simulink model "x_dd"  (R2020b)
settings: Solver=VariableStepAuto  StartTime=0.0  StopTime=10.0  RelTol=1e-3
settings Model: Creator=64200047  LastModifiedBy=64200047

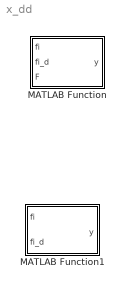
== system x_dd ==
  MATLAB Function : MATLAB Function  TreatAsAtomicUnit=on
  MATLAB Function1 : MATLAB Function  TreatAsAtomicUnit=on

== matlab function x_dd/MATLAB Function ==
  data: fi input; y output; fi_d input; F input
function y = fcn(fi, fi_d, F)
% x 

m1 = 2;
m2 = 0.31;
l = 0.5;

c1 = 1/(m1+m2);
k1 = +m2*l*sin(fi)*fi_d^2;
k2 = m2*l*cos(fi)*(cos(fi) + g*sin(fi));


y = c1*(k1+k2+F);

== matlab function x_dd/MATLAB Function1 ==
  data: fi input; y output; fi_d input
function y = fcn(fi, fi_d)
% fi

m1 = 2;
m2 = 0.31;
l = 0.5;
g = 9.81;

c1 = 1/(-(m2*l*cos(fi))^2*1/(m1+m2) + m2*l^2);

k1 = -m2*l*cos(fi)*1/(m1+m2) * (F + m2*l*sin(fi)*fi_d^2) - m2*g*l*sin(fi);


    
y = c1*k1;
